simulink model "IEEE39_IBR_FrequencyControl_Fullversion_2020a"  (R2020a)
settings: Solver=VariableStepAuto  StartTime=0.0  StopTime=30  RelTol=1e-3
InitFcn:
  | IEEE39data_FrencyControl_full_Opensource;
undefined symbols (not defined in the file): alpha, c, eps_ps, eps_u, Fref, IBR_data, line, Sbase, t_start_disturbance, t_startcontrol, Vbase
libraries: powerlib x202, powerlib_meascontrol x81, powerlib_extras x27, simulink x18
(part 4 of 5)

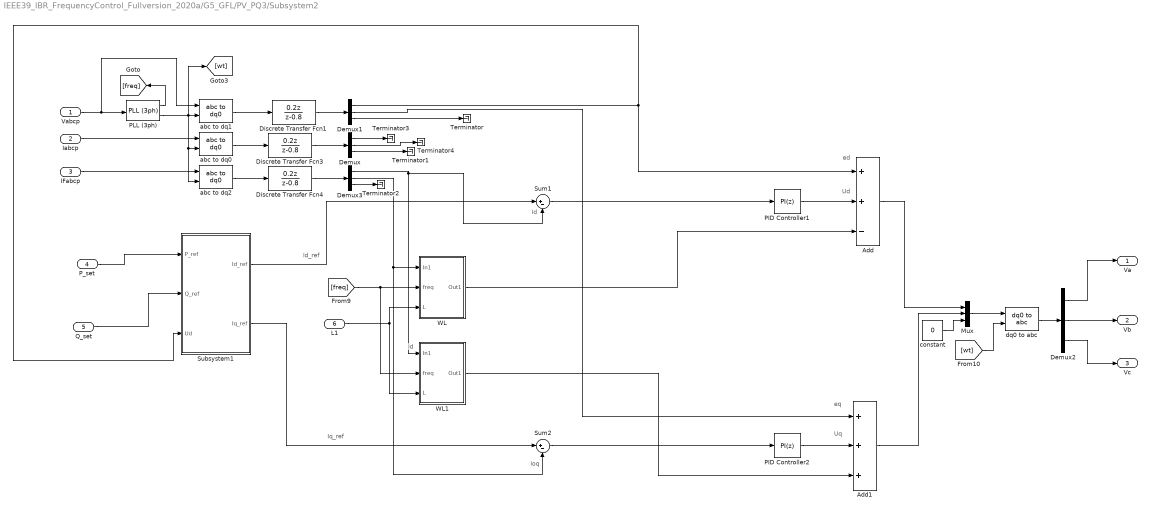
== system IEEE39_IBR_FrequencyControl_Fullversion_2020a/G5_GFL/PV_PQ3/Subsystem2 ==
  note: Iq_ref
  note: Id
  note: Id_ref
  note: Ud
  note: Uq
  note: eq
  note: ed
  note: Ioq
  note: Id
  Vabcp : Inport
  Iabcp : Inport  Port=2
  IFabcp : Inport  Port=3
  P_set : Inport  Port=4
  Q_set : Inport  Port=5
  L1 : Inport  Port=6
  Add : Sum  Inputs=++-
  Add1 : Sum  Inputs=+++
  Demux{,1..3} (4 alike) : Demux  Outputs=3
  Discrete Transfer Fcn1 : DiscreteTransferFcn  Numerator=[0.2 0]  Denominator=[1 -0.8]  InitialStates=[1 1 1]  SampleTime=5e-4
  Discrete Transfer Fcn3 : DiscreteTransferFcn  Numerator=[0.2 0]  Denominator=[1 -0.8]  SampleTime=5e-4
  Discrete Transfer Fcn4 : DiscreteTransferFcn  Numerator=[0.2 0]  Denominator=[1 -0.8]  SampleTime=5e-4
  Mux : Mux  Inputs=3
  PID Controller1 : simulink/Continuous/PID Controller  Controller=PI  Form=Parallel  TimeDomain=Discrete-time  UseExternalTs=off  SampleTime=5e-4  IntegratorMethod=Forward Euler  ControllerParametersSource=internal  P=100  I=400  D=0  N=100  UseFilter=on  TunerSelectOption=Transfer Function Based (PID Tuner App)  InitialConditionSource=internal  InitialConditionForIntegrator=0  InitialConditionForFilter=0  DifferentiatorICPrevScaledInput=0  ExternalReset=none  TrackingMode=off  Kt=1  LimitOutput=off  UpperSaturationLimit=inf  LowerSaturationLimit=-inf  LinearizeAsGain=on  AntiWindupMode=none  Kb=1  POutMin=[]  POutMax=[]  IOutMin=[]  IOutMax=[]  DOutMin=[]  DOutMax=[]  NOutMin=[]  NOutMax=[]  SumOutMin=[]  SumOutMax=[]  SaturationOutMin=[]  SaturationOutMax=[]  PParamMin=[]  PParamMax=[]  IParamMin=[]  IParamMax=[]  DParamMin=[]  DParamMax=[]  NParamMin=[]  NParamMax=[]  KbParamMin=[]  KbParamMax=[]  KtParamMin=[]  KtParamMax=[]  KbOutMin=[]  KbOutMax=[]  KtOutMin=[]  KtOutMax=[]  IntegratorOutMin=[]  IntegratorOutMax=[]  FilterOutMin=[]  FilterOutMax=[]  SumI1OutMin=[]  SumI1OutMax=[]  SumI2OutMin=[]  SumI2OutMax=[]  SumI3OutMin=[]  SumI3OutMax=[]  SumI4OutMin=[]  SumI4OutMax=[]  SumDOutMin=[]  SumDOutMax=[]  DifferentiatorOutMin=[]  DifferentiatorOutMax=[]  FilterDiffOutCoefMin=[]  FilterDiffOutCoefMax=[]  ReciprocalOutMin=[]  ReciprocalOutMax=[]  SumDenOutMin=[]  SumDenOutMax=[]  SumNumOutMin=[]  SumNumOutMax=[]  DivideOutMin=[]  DivideOutMax=[]  UdiffTsProdOutMin=[]  UdiffTsProdOutMax=[]  NTsProdOutMin=[]  NTsProdOutMax=[]  UintegralTsProdOutMin=[]  UintegralTsProdOutMax=[]  UngainTsProdOutMin=[]  UngainTsProdOutMax=[]  IntegratorContinuousStateAttributes=''  IntegratorStateMustResolveToSignalObject=off  IntegratorRTWStateStorageClass=Auto  FilterContinuousStateAttributes=''  FilterStateMustResolveToSignalObject=off  FilterRTWStateStorageClass=Auto  ParallelPVariant=InternalParameters  IdealPVariant=Disabled  IVariant=InternalParameters  DVariant=Disabled  IntegratorVariant=Discrete  SatVariant=Disabled  AWVariant=Passthrough  PCopyVariant=Disabled  TRVariant=Disabled  FdbkBlocksVariant=Forward  IdealPFdbkVariant=Disabled  SatFdbkVariant=Disabled  DerivativeFilterVariant=Disabled  NVariant=Disabled  NCopyVariant=Disabled_SignalSpec  FilterICVariant=Disabled  IntegratorICVariant=InternalICs  ExternalResetVariant=Disabled  TRSumVariant=Passthrough  SumFdbkVariant=Disabled  SumVariant=Sum_PI  TsampFilterVariant=InternalTs  TsampNgainVariant=Passthrough  TsampIntegralVariant=Disabled_SignalSpec
  PID Controller2 : simulink/Continuous/PID Controller  Controller=PI  Form=Parallel  TimeDomain=Discrete-time  UseExternalTs=off  SampleTime=5e-4  IntegratorMethod=Forward Euler  ControllerParametersSource=internal  P=100  I=400  D=0  N=100  UseFilter=on  TunerSelectOption=Transfer Function Based (PID Tuner App)  InitialConditionSource=internal  InitialConditionForIntegrator=0  InitialConditionForFilter=0  DifferentiatorICPrevScaledInput=0  ExternalReset=none  TrackingMode=off  Kt=1  LimitOutput=off  UpperSaturationLimit=inf  LowerSaturationLimit=-inf  LinearizeAsGain=on  AntiWindupMode=none  Kb=1  POutMin=[]  POutMax=[]  IOutMin=[]  IOutMax=[]  DOutMin=[]  DOutMax=[]  NOutMin=[]  NOutMax=[]  SumOutMin=[]  SumOutMax=[]  SaturationOutMin=[]  SaturationOutMax=[]  PParamMin=[]  PParamMax=[]  IParamMin=[]  IParamMax=[]  DParamMin=[]  DParamMax=[]  NParamMin=[]  NParamMax=[]  KbParamMin=[]  KbParamMax=[]  KtParamMin=[]  KtParamMax=[]  KbOutMin=[]  KbOutMax=[]  KtOutMin=[]  KtOutMax=[]  IntegratorOutMin=[]  IntegratorOutMax=[]  FilterOutMin=[]  FilterOutMax=[]  SumI1OutMin=[]  SumI1OutMax=[]  SumI2OutMin=[]  SumI2OutMax=[]  SumI3OutMin=[]  SumI3OutMax=[]  SumI4OutMin=[]  SumI4OutMax=[]  SumDOutMin=[]  SumDOutMax=[]  DifferentiatorOutMin=[]  DifferentiatorOutMax=[]  FilterDiffOutCoefMin=[]  FilterDiffOutCoefMax=[]  ReciprocalOutMin=[]  ReciprocalOutMax=[]  SumDenOutMin=[]  SumDenOutMax=[]  SumNumOutMin=[]  SumNumOutMax=[]  DivideOutMin=[]  DivideOutMax=[]  UdiffTsProdOutMin=[]  UdiffTsProdOutMax=[]  NTsProdOutMin=[]  NTsProdOutMax=[]  UintegralTsProdOutMin=[]  UintegralTsProdOutMax=[]  UngainTsProdOutMin=[]  UngainTsProdOutMax=[]  IntegratorContinuousStateAttributes=''  IntegratorStateMustResolveToSignalObject=off  IntegratorRTWStateStorageClass=Auto  FilterContinuousStateAttributes=''  FilterStateMustResolveToSignalObject=off  FilterRTWStateStorageClass=Auto  ParallelPVariant=InternalParameters  IdealPVariant=Disabled  IVariant=InternalParameters  DVariant=Disabled  IntegratorVariant=Discrete  SatVariant=Disabled  AWVariant=Passthrough  PCopyVariant=Disabled  TRVariant=Disabled  FdbkBlocksVariant=Forward  IdealPFdbkVariant=Disabled  SatFdbkVariant=Disabled  DerivativeFilterVariant=Disabled  NVariant=Disabled  NCopyVariant=Disabled_SignalSpec  FilterICVariant=Disabled  IntegratorICVariant=InternalICs  ExternalResetVariant=Disabled  TRSumVariant=Passthrough  SumFdbkVariant=Disabled  SumVariant=Sum_PI  TsampFilterVariant=InternalTs  TsampNgainVariant=Passthrough  TsampIntegralVariant=Disabled_SignalSpec
  PLL (3ph) : powerlib_meascontrol/PLL/PLL (3ph)  Fmin=59.5  Par_Init=[0, 60]  ParK=[180, 3200, 1]  TcD=1e-4  MaxRateChangeFreq=12  FilterCutOffFreq=25  Ts=1e-5  AGC=on
  Subsystem1 : Subsystem
  Sum1 : Sum  Inputs=|+-
  Sum2 : Sum  Inputs=|+-
  Terminator{,1..4} (5 alike) : Terminator
  WL : Subsystem
  WL1 : Subsystem
  abc to dq0 : powerlib_meascontrol/Transformations/abc to dq0  Alignment=90 degrees behind phase A axis
  abc to dq1 : powerlib_meascontrol/Transformations/abc to dq0  Alignment=90 degrees behind phase A axis
  abc to dq2 : powerlib_meascontrol/Transformations/abc to dq0  Alignment=90 degrees behind phase A axis
  constant : Constant  Value=0
  dq0 to abc : powerlib_meascontrol/Transformations/dq0 to abc  Alignment=90 degrees behind phase A axis
  Va : Outport  VectorParamsAs1DForOutWhenUnconnected=off
  Vb : Outport  Port=2  VectorParamsAs1DForOutWhenUnconnected=off
  Vc : Outport  Port=3  VectorParamsAs1DForOutWhenUnconnected=off
  wires:
  abc to dq0/1 -> Discrete Transfer Fcn3/1
  PLL (3ph)/2 -> [wt], abc to dq1/2, abc to dq2/2, abc to dq0/2
  Demux1/1 -> Add/1, Subsystem1/3(Ud)
  L1/1 -> WL/3(L), WL1/3(L)
  WL/1(Out1) -> Add/3
  [freq] -> WL1/2(freq), WL/2(freq)
  PLL (3ph)/1 -> [freq]
  Demux2/1 -> Va/1
  Add/1 -> Mux/1
  PID Controller2/1 -> Add1/2
  Demux2/2 -> Vb/1
  WL1/1(Out1) -> Add1/3
  Demux1/2 -> Add1/1
  Add1/1 -> Mux/2
  Mux/1 -> dq0 to abc/1
  Demux2/3 -> Vc/1
  dq0 to abc/1 -> Demux2/1
  Subsystem1/1(Id_ref) -> Sum1/1
  PID Controller1/1 -> Add/2
  [wt] -> dq0 to abc/2
  Subsystem1/2(Iq_ref) -> Sum2/1
  Demux1/3 -> Terminator/1
  Demux/3 -> Terminator1/1
  constant/1 -> Mux/3
  IFabcp/1 -> abc to dq2/1
  abc to dq2/1 -> Discrete Transfer Fcn4/1
  Demux3/3 -> Terminator2/1
  Demux3/2 -> Sum2/2, WL/1(In1)
  Demux3/1 -> Sum1/2, WL1/1(In1)
  Sum1/1 -> PID Controller1/1
  Sum2/1 -> PID Controller2/1
  P_set/1 -> Subsystem1/1(P_ref)
  Q_set/1 -> Subsystem1/2(Q_ref)
  Discrete Transfer Fcn3/1 -> Demux/1
  Discrete Transfer Fcn4/1 -> Demux3/1
  Demux/1 -> Terminator3/1
  Demux/2 -> Terminator4/1
  Discrete Transfer Fcn1/1 -> Demux1/1
  Iabcp/1 -> abc to dq0/1
  Vabcp/1 -> abc to dq1/1, PLL (3ph)/1
  abc to dq1/1 -> Discrete Transfer Fcn1/1

== system IEEE39_IBR_FrequencyControl_Fullversion_2020a/G6_GFL/PV_PQ3/Freq_Droop ==
  Pref : Inport
  Fref : Inport  Port=2
  Freq : Inport  Port=3
  D : Inport  Port=4
  Clock : Clock
  Constant : Constant  Value=0
  Divide : Product  Inputs=*/
  Product{,1..3} (4 alike) : Product
  S_base : Constant  Value=Sbase
  S_base1 : Constant  Value=Sbase
  Saturation : Saturate  UpperLimit=10*Sbase  LowerLimit=0  ZeroCross=off
  Subsystem : Subsystem
  Sum : Sum  Inputs=|+-
  Sum1 : Sum  Inputs=|+--
  Switch : Switch  Criteria=u2 > Threshold  Threshold=t_startcontrol  ZeroCross=off
  Transfer Fcn : TransferFcn  Denominator=[0.318 1]
  Pset : Outport
  tag scope: deltaP6=global
  wires:
  Freq/1 -> Sum/1
  Fref/1 -> Sum/2, Divide/2
  S_base/1 -> Product/2
  D/1 -> Product2/1, Product1/1
  Product/1 -> Product1/2
  Pref/1 -> Sum1/1
  Product1/1 -> Sum1/2
  Saturation/1 -> Pset/1
  Sum1/1 -> Saturation/1
  Subsystem/1(delatPset) -> Switch/1
  Clock/1 -> Switch/2
  Sum/1 -> Divide/1
  Constant/1 -> Switch/3
  Product2/1 -> Subsystem/1(Dw)
  Switch/1 -> [deltaP6], Product3/1
  S_base1/1 -> Product3/2
  Product3/1 -> Sum1/3
  Transfer Fcn/1 -> Subsystem/2(w), Product2/2, Product/1
  Divide/1 -> Transfer Fcn/1

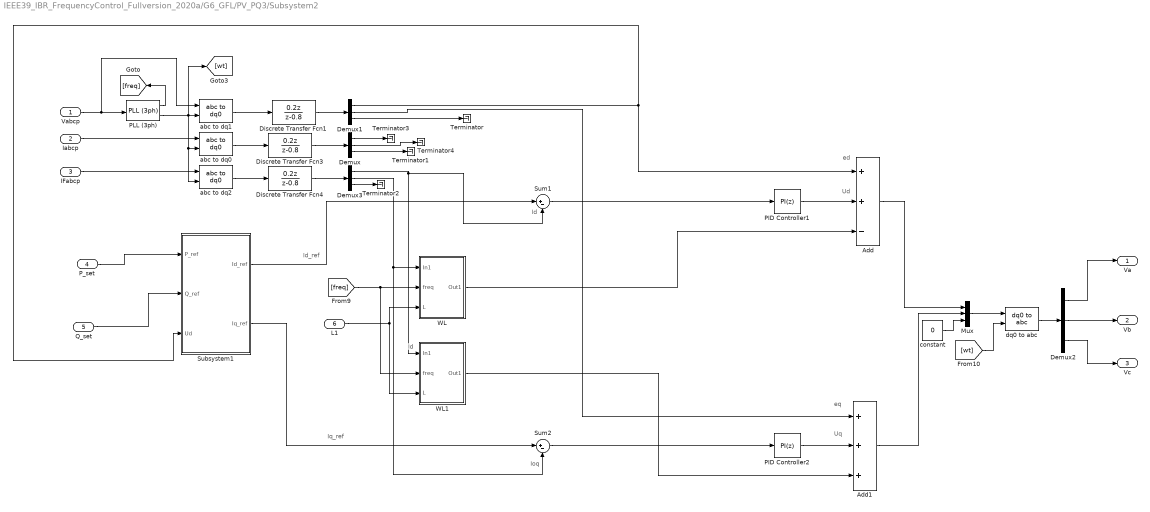
== system IEEE39_IBR_FrequencyControl_Fullversion_2020a/G6_GFL/PV_PQ3/Subsystem2 ==
  note: Iq_ref
  note: Id
  note: Id_ref
  note: Ud
  note: Uq
  note: eq
  note: ed
  note: Ioq
  note: Id
  Vabcp : Inport
  Iabcp : Inport  Port=2
  IFabcp : Inport  Port=3
  P_set : Inport  Port=4
  Q_set : Inport  Port=5
  L1 : Inport  Port=6
  Add : Sum  Inputs=++-
  Add1 : Sum  Inputs=+++
  Demux{,1..3} (4 alike) : Demux  Outputs=3
  Discrete Transfer Fcn1 : DiscreteTransferFcn  Numerator=[0.2 0]  Denominator=[1 -0.8]  InitialStates=[1 1 1]  SampleTime=5e-4
  Discrete Transfer Fcn3 : DiscreteTransferFcn  Numerator=[0.2 0]  Denominator=[1 -0.8]  SampleTime=5e-4
  Discrete Transfer Fcn4 : DiscreteTransferFcn  Numerator=[0.2 0]  Denominator=[1 -0.8]  SampleTime=5e-4
  Mux : Mux  Inputs=3
  PID Controller1 : simulink/Continuous/PID Controller  Controller=PI  Form=Parallel  TimeDomain=Discrete-time  UseExternalTs=off  SampleTime=5e-4  IntegratorMethod=Forward Euler  ControllerParametersSource=internal  P=50  I=400  D=0  N=100  UseFilter=on  TunerSelectOption=Transfer Function Based (PID Tuner App)  InitialConditionSource=internal  InitialConditionForIntegrator=0  InitialConditionForFilter=0  DifferentiatorICPrevScaledInput=0  ExternalReset=none  TrackingMode=off  Kt=1  LimitOutput=off  UpperSaturationLimit=inf  LowerSaturationLimit=-inf  LinearizeAsGain=on  AntiWindupMode=none  Kb=1  POutMin=[]  POutMax=[]  IOutMin=[]  IOutMax=[]  DOutMin=[]  DOutMax=[]  NOutMin=[]  NOutMax=[]  SumOutMin=[]  SumOutMax=[]  SaturationOutMin=[]  SaturationOutMax=[]  PParamMin=[]  PParamMax=[]  IParamMin=[]  IParamMax=[]  DParamMin=[]  DParamMax=[]  NParamMin=[]  NParamMax=[]  KbParamMin=[]  KbParamMax=[]  KtParamMin=[]  KtParamMax=[]  KbOutMin=[]  KbOutMax=[]  KtOutMin=[]  KtOutMax=[]  IntegratorOutMin=[]  IntegratorOutMax=[]  FilterOutMin=[]  FilterOutMax=[]  SumI1OutMin=[]  SumI1OutMax=[]  SumI2OutMin=[]  SumI2OutMax=[]  SumI3OutMin=[]  SumI3OutMax=[]  SumI4OutMin=[]  SumI4OutMax=[]  SumDOutMin=[]  SumDOutMax=[]  DifferentiatorOutMin=[]  DifferentiatorOutMax=[]  FilterDiffOutCoefMin=[]  FilterDiffOutCoefMax=[]  ReciprocalOutMin=[]  ReciprocalOutMax=[]  SumDenOutMin=[]  SumDenOutMax=[]  SumNumOutMin=[]  SumNumOutMax=[]  DivideOutMin=[]  DivideOutMax=[]  UdiffTsProdOutMin=[]  UdiffTsProdOutMax=[]  NTsProdOutMin=[]  NTsProdOutMax=[]  UintegralTsProdOutMin=[]  UintegralTsProdOutMax=[]  UngainTsProdOutMin=[]  UngainTsProdOutMax=[]  IntegratorContinuousStateAttributes=''  IntegratorStateMustResolveToSignalObject=off  IntegratorRTWStateStorageClass=Auto  FilterContinuousStateAttributes=''  FilterStateMustResolveToSignalObject=off  FilterRTWStateStorageClass=Auto  ParallelPVariant=InternalParameters  IdealPVariant=Disabled  IVariant=InternalParameters  DVariant=Disabled  IntegratorVariant=Discrete  SatVariant=Disabled  AWVariant=Passthrough  PCopyVariant=Disabled  TRVariant=Disabled  FdbkBlocksVariant=Forward  IdealPFdbkVariant=Disabled  SatFdbkVariant=Disabled  DerivativeFilterVariant=Disabled  NVariant=Disabled  NCopyVariant=Disabled_SignalSpec  FilterICVariant=Disabled  IntegratorICVariant=InternalICs  ExternalResetVariant=Disabled  TRSumVariant=Passthrough  SumFdbkVariant=Disabled  SumVariant=Sum_PI  TsampFilterVariant=InternalTs  TsampNgainVariant=Passthrough  TsampIntegralVariant=Disabled_SignalSpec
  PID Controller2 : simulink/Continuous/PID Controller  Controller=PI  Form=Parallel  TimeDomain=Discrete-time  UseExternalTs=off  SampleTime=5e-4  IntegratorMethod=Forward Euler  ControllerParametersSource=internal  P=50  I=400  D=0  N=100  UseFilter=on  TunerSelectOption=Transfer Function Based (PID Tuner App)  InitialConditionSource=internal  InitialConditionForIntegrator=0  InitialConditionForFilter=0  DifferentiatorICPrevScaledInput=0  ExternalReset=none  TrackingMode=off  Kt=1  LimitOutput=off  UpperSaturationLimit=inf  LowerSaturationLimit=-inf  LinearizeAsGain=on  AntiWindupMode=none  Kb=1  POutMin=[]  POutMax=[]  IOutMin=[]  IOutMax=[]  DOutMin=[]  DOutMax=[]  NOutMin=[]  NOutMax=[]  SumOutMin=[]  SumOutMax=[]  SaturationOutMin=[]  SaturationOutMax=[]  PParamMin=[]  PParamMax=[]  IParamMin=[]  IParamMax=[]  DParamMin=[]  DParamMax=[]  NParamMin=[]  NParamMax=[]  KbParamMin=[]  KbParamMax=[]  KtParamMin=[]  KtParamMax=[]  KbOutMin=[]  KbOutMax=[]  KtOutMin=[]  KtOutMax=[]  IntegratorOutMin=[]  IntegratorOutMax=[]  FilterOutMin=[]  FilterOutMax=[]  SumI1OutMin=[]  SumI1OutMax=[]  SumI2OutMin=[]  SumI2OutMax=[]  SumI3OutMin=[]  SumI3OutMax=[]  SumI4OutMin=[]  SumI4OutMax=[]  SumDOutMin=[]  SumDOutMax=[]  DifferentiatorOutMin=[]  DifferentiatorOutMax=[]  FilterDiffOutCoefMin=[]  FilterDiffOutCoefMax=[]  ReciprocalOutMin=[]  ReciprocalOutMax=[]  SumDenOutMin=[]  SumDenOutMax=[]  SumNumOutMin=[]  SumNumOutMax=[]  DivideOutMin=[]  DivideOutMax=[]  UdiffTsProdOutMin=[]  UdiffTsProdOutMax=[]  NTsProdOutMin=[]  NTsProdOutMax=[]  UintegralTsProdOutMin=[]  UintegralTsProdOutMax=[]  UngainTsProdOutMin=[]  UngainTsProdOutMax=[]  IntegratorContinuousStateAttributes=''  IntegratorStateMustResolveToSignalObject=off  IntegratorRTWStateStorageClass=Auto  FilterContinuousStateAttributes=''  FilterStateMustResolveToSignalObject=off  FilterRTWStateStorageClass=Auto  ParallelPVariant=InternalParameters  IdealPVariant=Disabled  IVariant=InternalParameters  DVariant=Disabled  IntegratorVariant=Discrete  SatVariant=Disabled  AWVariant=Passthrough  PCopyVariant=Disabled  TRVariant=Disabled  FdbkBlocksVariant=Forward  IdealPFdbkVariant=Disabled  SatFdbkVariant=Disabled  DerivativeFilterVariant=Disabled  NVariant=Disabled  NCopyVariant=Disabled_SignalSpec  FilterICVariant=Disabled  IntegratorICVariant=InternalICs  ExternalResetVariant=Disabled  TRSumVariant=Passthrough  SumFdbkVariant=Disabled  SumVariant=Sum_PI  TsampFilterVariant=InternalTs  TsampNgainVariant=Passthrough  TsampIntegralVariant=Disabled_SignalSpec
  PLL (3ph) : powerlib_meascontrol/PLL/PLL (3ph)  Fmin=59.5  Par_Init=[0, 60]  ParK=[180, 3200, 1]  TcD=1e-4  MaxRateChangeFreq=12  FilterCutOffFreq=25  Ts=1e-5  AGC=on
  Subsystem1 : Subsystem
  Sum1 : Sum  Inputs=|+-
  Sum2 : Sum  Inputs=|+-
  Terminator{,1..4} (5 alike) : Terminator
  WL : Subsystem
  WL1 : Subsystem
  abc to dq0 : powerlib_meascontrol/Transformations/abc to dq0  Alignment=90 degrees behind phase A axis
  abc to dq1 : powerlib_meascontrol/Transformations/abc to dq0  Alignment=90 degrees behind phase A axis
  abc to dq2 : powerlib_meascontrol/Transformations/abc to dq0  Alignment=90 degrees behind phase A axis
  constant : Constant  Value=0
  dq0 to abc : powerlib_meascontrol/Transformations/dq0 to abc  Alignment=90 degrees behind phase A axis
  Va : Outport  VectorParamsAs1DForOutWhenUnconnected=off
  Vb : Outport  Port=2  VectorParamsAs1DForOutWhenUnconnected=off
  Vc : Outport  Port=3  VectorParamsAs1DForOutWhenUnconnected=off
  wires:
  abc to dq0/1 -> Discrete Transfer Fcn3/1
  PLL (3ph)/2 -> [wt], abc to dq1/2, abc to dq2/2, abc to dq0/2
  Demux1/1 -> Add/1, Subsystem1/3(Ud)
  L1/1 -> WL/3(L), WL1/3(L)
  WL/1(Out1) -> Add/3
  [freq] -> WL1/2(freq), WL/2(freq)
  PLL (3ph)/1 -> [freq]
  Demux2/1 -> Va/1
  Add/1 -> Mux/1
  PID Controller2/1 -> Add1/2
  Demux2/2 -> Vb/1
  WL1/1(Out1) -> Add1/3
  Demux1/2 -> Add1/1
  Add1/1 -> Mux/2
  Mux/1 -> dq0 to abc/1
  Demux2/3 -> Vc/1
  dq0 to abc/1 -> Demux2/1
  Subsystem1/1(Id_ref) -> Sum1/1
  PID Controller1/1 -> Add/2
  [wt] -> dq0 to abc/2
  Subsystem1/2(Iq_ref) -> Sum2/1
  Demux1/3 -> Terminator/1
  Demux/3 -> Terminator1/1
  constant/1 -> Mux/3
  IFabcp/1 -> abc to dq2/1
  abc to dq2/1 -> Discrete Transfer Fcn4/1
  Demux3/3 -> Terminator2/1
  Demux3/2 -> Sum2/2, WL/1(In1)
  Demux3/1 -> Sum1/2, WL1/1(In1)
  Sum1/1 -> PID Controller1/1
  Sum2/1 -> PID Controller2/1
  P_set/1 -> Subsystem1/1(P_ref)
  Q_set/1 -> Subsystem1/2(Q_ref)
  Discrete Transfer Fcn3/1 -> Demux/1
  Discrete Transfer Fcn4/1 -> Demux3/1
  Demux/1 -> Terminator3/1
  Demux/2 -> Terminator4/1
  Discrete Transfer Fcn1/1 -> Demux1/1
  Iabcp/1 -> abc to dq0/1
  Vabcp/1 -> abc to dq1/1, PLL (3ph)/1
  abc to dq1/1 -> Discrete Transfer Fcn1/1

== system IEEE39_IBR_FrequencyControl_Fullversion_2020a/GFM1/PV_PQ3/Freq_Droop ==
  Pref : Inport
  Fref : Inport  Port=2
  Pmeans : Inport  Port=3
  Add : Sum  Inputs=+-
  Add1 : Sum
  Add2 : Sum  Inputs=+-
  Add3 : Sum  Inputs=+-
  Divide : Product  Inputs=*/
  Divide2 : Product  Inputs=*/
  Product : Product
  S_base : Constant  Value=Sbase
  Saturation : Saturate  UpperLimit=2  LowerLimit=-2  ZeroCross=off
  Step : Step  Time=5  SampleTime=0
  Subsystem1 : Subsystem
  Switch : Switch  Criteria=u2 > Threshold
  Transfer Fcn : TransferFcn  Denominator=[IBR_data(10,5) IBR_data(10,4)]
  Transfer Fcn1 : TransferFcn  Numerator=[20]  Denominator=[1 20]
  Transfer Fcn2 : TransferFcn  Denominator=[IBR_data(10,5) IBR_data(10,4)]
  fset : Outport
  wires:
  Pref/1 -> Add/1
  Transfer Fcn1/1 -> Add/2
  S_base/1 -> Divide/2
  Switch/1 -> Product/1
  Add1/1 -> fset/1
  Saturation/1 -> Add1/1
  Product/1 -> Saturation/1
  Divide/1 -> Add3/1
  Add/1 -> Divide/1
  Pmeans/1 -> Transfer Fcn1/1
  [f10] -> Add2/1
  Fref/1 -> Add1/2, Divide2/2, Add2/2, Product/2
  Add2/1 -> Divide2/1
  Divide2/1 -> Subsystem1/1(w)
  Transfer Fcn2/1 -> Switch/1
  Transfer Fcn/1 -> Switch/3
  Step/1 -> Switch/2
  Add3/1 -> Transfer Fcn/1, Transfer Fcn2/1
  Subsystem1/1(Out1) -> Add3/2

== system IEEE39_IBR_FrequencyControl_Fullversion_2020a/GFM1/PV_PQ3/V//F ==
  vabcb : Inport
  iabcb : Inport  Port=2
  iFabcb : Inport  Port=3
  Vref_LL : Inport  Port=4
  f : Inport  Port=5
  Init_Phase_degree : Inport  Port=6
  Constant1 : Constant  Value=0
  Constant2 : Constant  Value=sqrt(2)/sqrt(3)
  Product : Product
  Subsystem : Subsystem
  UIcontrol : Subsystem
  Va : Outport
  Vb : Outport  Port=2
  Vc : Outport  Port=3
  wires:
  Constant1/1 -> UIcontrol/3(eq_ref)
  vabcb/1 -> Subsystem/1(eo)
  iFabcb/1 -> Subsystem/3(i)
  iabcb/1 -> Subsystem/2(io)
  Subsystem/1(eod) -> UIcontrol/2(ed)
  Subsystem/2(eoq) -> UIcontrol/4(eq)
  Subsystem/3(iod) -> UIcontrol/5(iod)
  Subsystem/4(ioq) -> UIcontrol/6(ioq)
  Subsystem/5(id) -> UIcontrol/7(id)
  Subsystem/6(iq) -> UIcontrol/8(iq)
  Subsystem/7(w) -> UIcontrol/9(w)
  UIcontrol/1(Va) -> Va/1
  UIcontrol/2(Vb) -> Vb/1
  UIcontrol/3(Vc) -> Vc/1
  f/1 -> Subsystem/4(f)
  Init_Phase_degree/1 -> Subsystem/5(Init_Phase_degree)
  Vref_LL/1 -> Product/1
  Product/1 -> UIcontrol/1(ed_ref)
  Constant2/1 -> Product/2
  Subsystem/8("wt ") -> UIcontrol/10("wt ")

== system IEEE39_IBR_FrequencyControl_Fullversion_2020a/GFM2/PV_PQ3/Freq_Droop ==
  Pref : Inport
  Fref : Inport  Port=2
  Pmeans : Inport  Port=3
  Add : Sum  Inputs=+-
  Add1 : Sum
  Add2 : Sum  Inputs=+-
  Add3 : Sum  Inputs=+-
  Divide : Product  Inputs=*/
  Divide2 : Product  Inputs=*/
  Product : Product
  S_base : Constant  Value=Sbase
  Saturation : Saturate  UpperLimit=2  LowerLimit=-2  ZeroCross=off
  Step : Step  Time=5  SampleTime=0
  Subsystem1 : Subsystem
  Switch : Switch  Criteria=u2 > Threshold
  Transfer Fcn : TransferFcn  Denominator=[IBR_data(9,5) IBR_data(9,4)]
  Transfer Fcn1 : TransferFcn  Numerator=[20]  Denominator=[1 20]
  Transfer Fcn2 : TransferFcn  Denominator=[IBR_data(9,5) IBR_data(9,4)]
  fset : Outport
  wires:
  Pref/1 -> Add/1
  Transfer Fcn1/1 -> Add/2
  S_base/1 -> Divide/2
  Switch/1 -> Product/1
  Add1/1 -> fset/1
  Saturation/1 -> Add1/1
  Product/1 -> Saturation/1
  Divide/1 -> Add3/1
  Add/1 -> Divide/1
  Pmeans/1 -> Transfer Fcn1/1
  [f9] -> Add2/1
  Fref/1 -> Add1/2, Divide2/2, Add2/2, Product/2
  Add2/1 -> Divide2/1
  Divide2/1 -> Subsystem1/1(w)
  Transfer Fcn2/1 -> Switch/1
  Transfer Fcn/1 -> Switch/3
  Step/1 -> Switch/2
  Add3/1 -> Transfer Fcn/1, Transfer Fcn2/1
  Subsystem1/1(Out1) -> Add3/2

== system IEEE39_IBR_FrequencyControl_Fullversion_2020a/GFM2/PV_PQ3/V//F ==
  vabcb : Inport
  iabcb : Inport  Port=2
  iFabcb : Inport  Port=3
  Vref_LL : Inport  Port=4
  f : Inport  Port=5
  Init_Phase_degree : Inport  Port=6
  Constant : Constant  Value=2*pi
  Constant1 : Constant  Value=0
  Constant2 : Constant  Value=sqrt(2)/sqrt(3)
  Divide : Product  Inputs=*/
  Product : Product
  Scope1 : Scope
  Subsystem : Subsystem
  UIcontrol : Subsystem
  Va : Outport
  Vb : Outport  Port=2
  Vc : Outport  Port=3
  wires:
  Constant1/1 -> UIcontrol/3(eq_ref)
  vabcb/1 -> Subsystem/1(eo)
  iFabcb/1 -> Subsystem/3(i)
  iabcb/1 -> Subsystem/2(io)
  Subsystem/1(eod) -> UIcontrol/2(ed)
  Subsystem/2(eoq) -> UIcontrol/4(eq)
  Subsystem/3(iod) -> UIcontrol/5(iod)
  Subsystem/4(ioq) -> UIcontrol/6(ioq)
  Subsystem/5(id) -> UIcontrol/7(id)
  Subsystem/6(iq) -> UIcontrol/8(iq)
  Subsystem/7(w) -> Divide/1, UIcontrol/9(w)
  UIcontrol/1(Va) -> Va/1
  UIcontrol/2(Vb) -> Vb/1
  UIcontrol/3(Vc) -> Vc/1
  f/1 -> Subsystem/4(f)
  Init_Phase_degree/1 -> Subsystem/5(Init_Phase_degree)
  Vref_LL/1 -> Product/1
  Product/1 -> UIcontrol/1(ed_ref)
  Constant2/1 -> Product/2
  Subsystem/8("wt ") -> UIcontrol/10("wt ")
  Constant/1 -> Divide/2
  Divide/1 -> Scope1/1

== system IEEE39_IBR_FrequencyControl_Fullversion_2020a/GFM3/PV_PQ3/Freq_Droop ==
  Pref : Inport
  Fref : Inport  Port=2
  Pmeans : Inport  Port=3
  Add : Sum  Inputs=+-
  Add1 : Sum
  Add2 : Sum  Inputs=+-
  Add3 : Sum  Inputs=+-
  Divide : Product  Inputs=*/
  Divide2 : Product  Inputs=*/
  Product : Product
  S_base : Constant  Value=Sbase
  Saturation : Saturate  UpperLimit=2  LowerLimit=-2  ZeroCross=off
  Step : Step  Time=5  SampleTime=0
  Subsystem1 : Subsystem
  Switch : Switch  Criteria=u2 > Threshold
  Transfer Fcn : TransferFcn  Denominator=[IBR_data(8,5) IBR_data(8,4)]
  Transfer Fcn1 : TransferFcn  Numerator=[20]  Denominator=[1 20]
  Transfer Fcn2 : TransferFcn  Denominator=[IBR_data(8,5) IBR_data(8,4)]
  fset : Outport
  wires:
  Pref/1 -> Add/1
  Transfer Fcn1/1 -> Add/2
  S_base/1 -> Divide/2
  Switch/1 -> Product/1
  Add1/1 -> fset/1
  Saturation/1 -> Add1/1
  Product/1 -> Saturation/1
  Divide/1 -> Add3/1
  Add/1 -> Divide/1
  Pmeans/1 -> Transfer Fcn1/1
  [f8] -> Add2/1
  Fref/1 -> Add1/2, Divide2/2, Add2/2, Product/2
  Add2/1 -> Divide2/1
  Divide2/1 -> Subsystem1/1(w)
  Transfer Fcn2/1 -> Switch/1
  Transfer Fcn/1 -> Switch/3
  Step/1 -> Switch/2
  Add3/1 -> Transfer Fcn/1, Transfer Fcn2/1
  Subsystem1/1(Out1) -> Add3/2

== system IEEE39_IBR_FrequencyControl_Fullversion_2020a/GFM3/PV_PQ3/V//F ==
  vabcb : Inport
  iabcb : Inport  Port=2
  iFabcb : Inport  Port=3
  Vref_LL : Inport  Port=4
  f : Inport  Port=5
  Init_Phase_degree : Inport  Port=6
  Constant : Constant  Value=2*pi
  Constant1 : Constant  Value=0
  Constant2 : Constant  Value=sqrt(2)/sqrt(3)
  Divide : Product  Inputs=*/
  Product : Product
  Scope1 : Scope
  Subsystem : Subsystem
  UIcontrol : Subsystem
  Va : Outport
  Vb : Outport  Port=2
  Vc : Outport  Port=3
  wires:
  Constant1/1 -> UIcontrol/3(eq_ref)
  vabcb/1 -> Subsystem/1(eo)
  iFabcb/1 -> Subsystem/3(i)
  iabcb/1 -> Subsystem/2(io)
  Subsystem/1(eod) -> UIcontrol/2(ed)
  Subsystem/2(eoq) -> UIcontrol/4(eq)
  Subsystem/3(iod) -> UIcontrol/5(iod)
  Subsystem/4(ioq) -> UIcontrol/6(ioq)
  Subsystem/5(id) -> UIcontrol/7(id)
  Subsystem/6(iq) -> UIcontrol/8(iq)
  Subsystem/7(w) -> Divide/1, UIcontrol/9(w)
  UIcontrol/1(Va) -> Va/1
  UIcontrol/2(Vb) -> Vb/1
  UIcontrol/3(Vc) -> Vc/1
  f/1 -> Subsystem/4(f)
  Init_Phase_degree/1 -> Subsystem/5(Init_Phase_degree)
  Vref_LL/1 -> Product/1
  Product/1 -> UIcontrol/1(ed_ref)
  Constant2/1 -> Product/2
  Subsystem/8("wt ") -> UIcontrol/10("wt ")
  Constant/1 -> Divide/2
  Divide/1 -> Scope1/1

== system IEEE39_IBR_FrequencyControl_Fullversion_2020a/GFM4/PV_PQ3/Freq_Droop ==
  Pref : Inport
  Fref : Inport  Port=2
  Pmeans : Inport  Port=3
  Add : Sum  Inputs=+-
  Add1 : Sum
  Add2 : Sum  Inputs=+-
  Add3 : Sum  Inputs=+-
  Divide : Product  Inputs=*/
  Divide2 : Product  Inputs=*/
  Product : Product
  S_base : Constant  Value=Sbase
  Saturation : Saturate  UpperLimit=2  LowerLimit=-2  ZeroCross=off
  Step : Step  Time=5  SampleTime=0
  Subsystem1 : Subsystem
  Switch : Switch  Criteria=u2 > Threshold
  Transfer Fcn : TransferFcn  Denominator=[IBR_data(7,5) IBR_data(7,4)]
  Transfer Fcn1 : TransferFcn  Numerator=[20]  Denominator=[1 20]
  Transfer Fcn2 : TransferFcn  Denominator=[IBR_data(7,5) IBR_data(7,4)]
  fset : Outport
  wires:
  Pref/1 -> Add/1
  Transfer Fcn1/1 -> Add/2
  S_base/1 -> Divide/2
  Switch/1 -> Product/1
  Add1/1 -> fset/1
  Saturation/1 -> Add1/1
  Product/1 -> Saturation/1
  Divide/1 -> Add3/1
  Add/1 -> Divide/1
  Pmeans/1 -> Transfer Fcn1/1
  [f8] -> Add2/1
  Fref/1 -> Add1/2, Divide2/2, Add2/2, Product/2
  Add2/1 -> Divide2/1
  Divide2/1 -> Subsystem1/1(w)
  Transfer Fcn2/1 -> Switch/1
  Transfer Fcn/1 -> Switch/3
  Step/1 -> Switch/2
  Add3/1 -> Transfer Fcn/1, Transfer Fcn2/1
  Subsystem1/1(Out1) -> Add3/2

== system IEEE39_IBR_FrequencyControl_Fullversion_2020a/GFM4/PV_PQ3/V//F ==
  vabcb : Inport
  iabcb : Inport  Port=2
  iFabcb : Inport  Port=3
  Vref_LL : Inport  Port=4
  f : Inport  Port=5
  Init_Phase_degree : Inport  Port=6
  Constant : Constant  Value=2*pi
  Constant1 : Constant  Value=0
  Constant2 : Constant  Value=sqrt(2)/sqrt(3)
  Divide : Product  Inputs=*/
  Product : Product
  Scope1 : Scope
  Subsystem : Subsystem
  UIcontrol : Subsystem
  Va : Outport
  Vb : Outport  Port=2
  Vc : Outport  Port=3
  wires:
  Constant1/1 -> UIcontrol/3(eq_ref)
  vabcb/1 -> Subsystem/1(eo)
  iFabcb/1 -> Subsystem/3(i)
  iabcb/1 -> Subsystem/2(io)
  Subsystem/1(eod) -> UIcontrol/2(ed)
  Subsystem/2(eoq) -> UIcontrol/4(eq)
  Subsystem/3(iod) -> UIcontrol/5(iod)
  Subsystem/4(ioq) -> UIcontrol/6(ioq)
  Subsystem/5(id) -> UIcontrol/7(id)
  Subsystem/6(iq) -> UIcontrol/8(iq)
  Subsystem/7(w) -> Divide/1, UIcontrol/9(w)
  UIcontrol/1(Va) -> Va/1
  UIcontrol/2(Vb) -> Vb/1
  UIcontrol/3(Vc) -> Vc/1
  f/1 -> Subsystem/4(f)
  Init_Phase_degree/1 -> Subsystem/5(Init_Phase_degree)
  Vref_LL/1 -> Product/1
  Product/1 -> UIcontrol/1(ed_ref)
  Constant2/1 -> Product/2
  Subsystem/8("wt ") -> UIcontrol/10("wt ")
  Constant/1 -> Divide/2
  Divide/1 -> Scope1/1

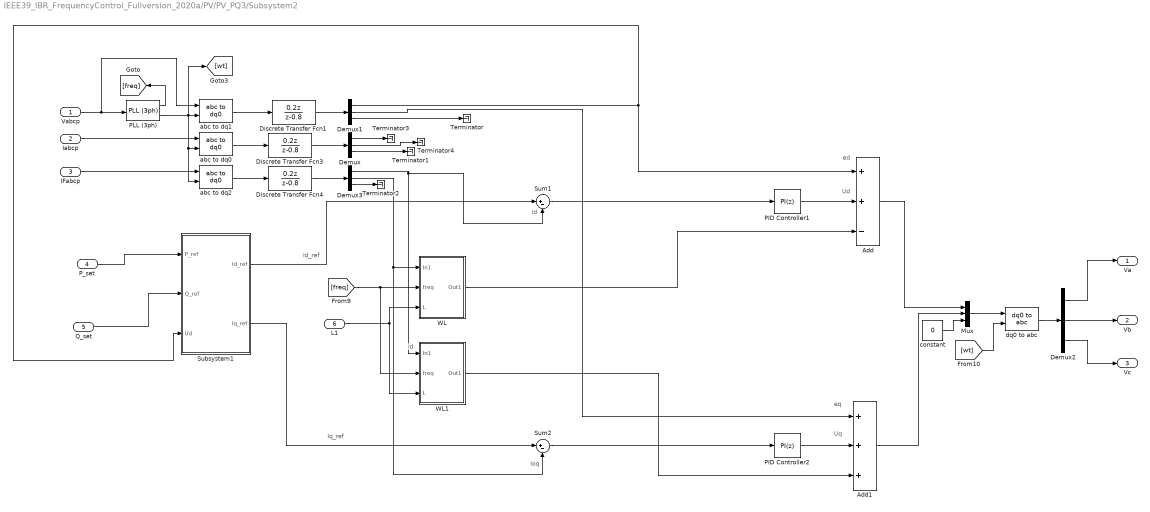
== system IEEE39_IBR_FrequencyControl_Fullversion_2020a/PV/PV_PQ3/Subsystem2 ==
  note: Iq_ref
  note: Id
  note: Id_ref
  note: Ud
  note: Uq
  note: eq
  note: ed
  note: Ioq
  note: Id
  Vabcp : Inport
  Iabcp : Inport  Port=2
  IFabcp : Inport  Port=3
  P_set : Inport  Port=4
  Q_set : Inport  Port=5
  L1 : Inport  Port=6
  Add : Sum  Inputs=++-
  Add1 : Sum  Inputs=+++
  Demux{,1..3} (4 alike) : Demux  Outputs=3
  Discrete Transfer Fcn1 : DiscreteTransferFcn  Numerator=[0.2 0]  Denominator=[1 -0.8]  InitialStates=[1 1 1]  SampleTime=5e-4
  Discrete Transfer Fcn3 : DiscreteTransferFcn  Numerator=[0.2 0]  Denominator=[1 -0.8]  SampleTime=5e-4
  Discrete Transfer Fcn4 : DiscreteTransferFcn  Numerator=[0.2 0]  Denominator=[1 -0.8]  SampleTime=5e-4
  Mux : Mux  Inputs=3
  PID Controller1 : simulink/Continuous/PID Controller  Controller=PI  Form=Parallel  TimeDomain=Discrete-time  UseExternalTs=off  SampleTime=5e-4  IntegratorMethod=Forward Euler  ControllerParametersSource=internal  P=100  I=400  D=0  N=100  UseFilter=on  TunerSelectOption=Transfer Function Based (PID Tuner App)  InitialConditionSource=internal  InitialConditionForIntegrator=0  InitialConditionForFilter=0  DifferentiatorICPrevScaledInput=0  ExternalReset=none  TrackingMode=off  Kt=1  LimitOutput=off  UpperSaturationLimit=inf  LowerSaturationLimit=-inf  LinearizeAsGain=on  AntiWindupMode=none  Kb=1  POutMin=[]  POutMax=[]  IOutMin=[]  IOutMax=[]  DOutMin=[]  DOutMax=[]  NOutMin=[]  NOutMax=[]  SumOutMin=[]  SumOutMax=[]  SaturationOutMin=[]  SaturationOutMax=[]  PParamMin=[]  PParamMax=[]  IParamMin=[]  IParamMax=[]  DParamMin=[]  DParamMax=[]  NParamMin=[]  NParamMax=[]  KbParamMin=[]  KbParamMax=[]  KtParamMin=[]  KtParamMax=[]  KbOutMin=[]  KbOutMax=[]  KtOutMin=[]  KtOutMax=[]  IntegratorOutMin=[]  IntegratorOutMax=[]  FilterOutMin=[]  FilterOutMax=[]  SumI1OutMin=[]  SumI1OutMax=[]  SumI2OutMin=[]  SumI2OutMax=[]  SumI3OutMin=[]  SumI3OutMax=[]  SumI4OutMin=[]  SumI4OutMax=[]  SumDOutMin=[]  SumDOutMax=[]  DifferentiatorOutMin=[]  DifferentiatorOutMax=[]  FilterDiffOutCoefMin=[]  FilterDiffOutCoefMax=[]  ReciprocalOutMin=[]  ReciprocalOutMax=[]  SumDenOutMin=[]  SumDenOutMax=[]  SumNumOutMin=[]  SumNumOutMax=[]  DivideOutMin=[]  DivideOutMax=[]  UdiffTsProdOutMin=[]  UdiffTsProdOutMax=[]  NTsProdOutMin=[]  NTsProdOutMax=[]  UintegralTsProdOutMin=[]  UintegralTsProdOutMax=[]  UngainTsProdOutMin=[]  UngainTsProdOutMax=[]  IntegratorContinuousStateAttributes=''  IntegratorStateMustResolveToSignalObject=off  IntegratorRTWStateStorageClass=Auto  FilterContinuousStateAttributes=''  FilterStateMustResolveToSignalObject=off  FilterRTWStateStorageClass=Auto  ParallelPVariant=InternalParameters  IdealPVariant=Disabled  IVariant=InternalParameters  DVariant=Disabled  IntegratorVariant=Discrete  SatVariant=Disabled  AWVariant=Passthrough  PCopyVariant=Disabled  TRVariant=Disabled  FdbkBlocksVariant=Forward  IdealPFdbkVariant=Disabled  SatFdbkVariant=Disabled  DerivativeFilterVariant=Disabled  NVariant=Disabled  NCopyVariant=Disabled_SignalSpec  FilterICVariant=Disabled  IntegratorICVariant=InternalICs  ExternalResetVariant=Disabled  TRSumVariant=Passthrough  SumFdbkVariant=Disabled  SumVariant=Sum_PI  TsampFilterVariant=InternalTs  TsampNgainVariant=Passthrough  TsampIntegralVariant=Disabled_SignalSpec
  PID Controller2 : simulink/Continuous/PID Controller  Controller=PI  Form=Parallel  TimeDomain=Discrete-time  UseExternalTs=off  SampleTime=5e-4  IntegratorMethod=Forward Euler  ControllerParametersSource=internal  P=100  I=400  D=0  N=100  UseFilter=on  TunerSelectOption=Transfer Function Based (PID Tuner App)  InitialConditionSource=internal  InitialConditionForIntegrator=0  InitialConditionForFilter=0  DifferentiatorICPrevScaledInput=0  ExternalReset=none  TrackingMode=off  Kt=1  LimitOutput=off  UpperSaturationLimit=inf  LowerSaturationLimit=-inf  LinearizeAsGain=on  AntiWindupMode=none  Kb=1  POutMin=[]  POutMax=[]  IOutMin=[]  IOutMax=[]  DOutMin=[]  DOutMax=[]  NOutMin=[]  NOutMax=[]  SumOutMin=[]  SumOutMax=[]  SaturationOutMin=[]  SaturationOutMax=[]  PParamMin=[]  PParamMax=[]  IParamMin=[]  IParamMax=[]  DParamMin=[]  DParamMax=[]  NParamMin=[]  NParamMax=[]  KbParamMin=[]  KbParamMax=[]  KtParamMin=[]  KtParamMax=[]  KbOutMin=[]  KbOutMax=[]  KtOutMin=[]  KtOutMax=[]  IntegratorOutMin=[]  IntegratorOutMax=[]  FilterOutMin=[]  FilterOutMax=[]  SumI1OutMin=[]  SumI1OutMax=[]  SumI2OutMin=[]  SumI2OutMax=[]  SumI3OutMin=[]  SumI3OutMax=[]  SumI4OutMin=[]  SumI4OutMax=[]  SumDOutMin=[]  SumDOutMax=[]  DifferentiatorOutMin=[]  DifferentiatorOutMax=[]  FilterDiffOutCoefMin=[]  FilterDiffOutCoefMax=[]  ReciprocalOutMin=[]  ReciprocalOutMax=[]  SumDenOutMin=[]  SumDenOutMax=[]  SumNumOutMin=[]  SumNumOutMax=[]  DivideOutMin=[]  DivideOutMax=[]  UdiffTsProdOutMin=[]  UdiffTsProdOutMax=[]  NTsProdOutMin=[]  NTsProdOutMax=[]  UintegralTsProdOutMin=[]  UintegralTsProdOutMax=[]  UngainTsProdOutMin=[]  UngainTsProdOutMax=[]  IntegratorContinuousStateAttributes=''  IntegratorStateMustResolveToSignalObject=off  IntegratorRTWStateStorageClass=Auto  FilterContinuousStateAttributes=''  FilterStateMustResolveToSignalObject=off  FilterRTWStateStorageClass=Auto  ParallelPVariant=InternalParameters  IdealPVariant=Disabled  IVariant=InternalParameters  DVariant=Disabled  IntegratorVariant=Discrete  SatVariant=Disabled  AWVariant=Passthrough  PCopyVariant=Disabled  TRVariant=Disabled  FdbkBlocksVariant=Forward  IdealPFdbkVariant=Disabled  SatFdbkVariant=Disabled  DerivativeFilterVariant=Disabled  NVariant=Disabled  NCopyVariant=Disabled_SignalSpec  FilterICVariant=Disabled  IntegratorICVariant=InternalICs  ExternalResetVariant=Disabled  TRSumVariant=Passthrough  SumFdbkVariant=Disabled  SumVariant=Sum_PI  TsampFilterVariant=InternalTs  TsampNgainVariant=Passthrough  TsampIntegralVariant=Disabled_SignalSpec
  PLL (3ph) : powerlib_meascontrol/PLL/PLL (3ph)  Fmin=59.5  Par_Init=[0, 60]  ParK=[180, 3200, 1]  TcD=1e-4  MaxRateChangeFreq=12  FilterCutOffFreq=25  Ts=1e-5  AGC=on
  Subsystem1 : Subsystem
  Sum1 : Sum  Inputs=|+-
  Sum2 : Sum  Inputs=|+-
  Terminator{,1..4} (5 alike) : Terminator
  WL : Subsystem
  WL1 : Subsystem
  abc to dq0 : powerlib_meascontrol/Transformations/abc to dq0  Alignment=90 degrees behind phase A axis
  abc to dq1 : powerlib_meascontrol/Transformations/abc to dq0  Alignment=90 degrees behind phase A axis
  abc to dq2 : powerlib_meascontrol/Transformations/abc to dq0  Alignment=90 degrees behind phase A axis
  constant : Constant  Value=0
  dq0 to abc : powerlib_meascontrol/Transformations/dq0 to abc  Alignment=90 degrees behind phase A axis
  Va : Outport  VectorParamsAs1DForOutWhenUnconnected=off
  Vb : Outport  Port=2  VectorParamsAs1DForOutWhenUnconnected=off
  Vc : Outport  Port=3  VectorParamsAs1DForOutWhenUnconnected=off
  wires:
  abc to dq0/1 -> Discrete Transfer Fcn3/1
  PLL (3ph)/2 -> [wt], abc to dq1/2, abc to dq2/2, abc to dq0/2
  Demux1/1 -> Add/1, Subsystem1/3(Ud)
  L1/1 -> WL/3(L), WL1/3(L)
  WL/1(Out1) -> Add/3
  [freq] -> WL1/2(freq), WL/2(freq)
  PLL (3ph)/1 -> [freq]
  Demux2/1 -> Va/1
  Add/1 -> Mux/1
  PID Controller2/1 -> Add1/2
  Demux2/2 -> Vb/1
  WL1/1(Out1) -> Add1/3
  Demux1/2 -> Add1/1
  Add1/1 -> Mux/2
  Mux/1 -> dq0 to abc/1
  Demux2/3 -> Vc/1
  dq0 to abc/1 -> Demux2/1
  Subsystem1/1(Id_ref) -> Sum1/1
  PID Controller1/1 -> Add/2
  [wt] -> dq0 to abc/2
  Subsystem1/2(Iq_ref) -> Sum2/1
  Demux1/3 -> Terminator/1
  Demux/3 -> Terminator1/1
  constant/1 -> Mux/3
  IFabcp/1 -> abc to dq2/1
  abc to dq2/1 -> Discrete Transfer Fcn4/1
  Demux3/3 -> Terminator2/1
  Demux3/2 -> Sum2/2, WL/1(In1)
  Demux3/1 -> Sum1/2, WL1/1(In1)
  Sum1/1 -> PID Controller1/1
  Sum2/1 -> PID Controller2/1
  P_set/1 -> Subsystem1/1(P_ref)
  Q_set/1 -> Subsystem1/2(Q_ref)
  Discrete Transfer Fcn3/1 -> Demux/1
  Discrete Transfer Fcn4/1 -> Demux3/1
  Demux/1 -> Terminator3/1
  Demux/2 -> Terminator4/1
  Discrete Transfer Fcn1/1 -> Demux1/1
  Iabcp/1 -> abc to dq0/1
  Vabcp/1 -> abc to dq1/1, PLL (3ph)/1
  abc to dq1/1 -> Discrete Transfer Fcn1/1

== system IEEE39_IBR_FrequencyControl_Fullversion_2020a/G1_GFL/PV_PQ3/Freq_Droop/Subsystem ==
  Dw : Inport
  w : Inport  Port=2
  Add1 : Sum
  Add2 : Sum  Inputs=+++
  Add3 : Sum  Inputs=-+
  Gain : Gain  Gain=eps_u
  Gain1 : Gain  Gain=eps_ps
  Gain2 : Gain  Gain=c(1)
  Gain3 : Gain  Gain=alpha
  Integrator : Integrator  ExternalReset=rising  ZeroCross=off
  Integrator1 : Integrator  ExternalReset=rising  ZeroCross=off
  Saturation : Saturate  UpperLimit=IBR_data(1,6)-IBR_data(1,10)  LowerLimit=IBR_data(1,6)-IBR_data(1,9)
  Scope : Scope  NumInputPorts=3
  Step : Step  Time=3  SampleTime=0
  Step1 : Step  Time=3  SampleTime=0
  delatPset : Outport
  wires:
  Gain2/1 -> Scope/1, Add2/1
  Integrator1/1 -> delatPset/1, Add3/1, Add1/1, Gain2/1
  Step/1 -> Integrator1/2
  Step1/1 -> Integrator/2
  Integrator/1 -> Gain/1
  Gain/1 -> Scope/3, Add2/2
  Dw/1 -> Integrator/1
  Gain1/1 -> Integrator1/1
  Add2/1 -> Gain3/1
  Gain3/1 -> Add1/2
  Add1/1 -> Saturation/1
  Saturation/1 -> Add3/2
  Add3/1 -> Gain1/1
  w/1 -> Scope/2, Add2/3

== system IEEE39_IBR_FrequencyControl_Fullversion_2020a/G1_GFL/PV_PQ3/Subsystem2/Subsystem1 ==
  P_ref : Inport
  Q_ref : Inport  Port=2
  Ud : Inport  Port=3
  Divide5 : Product  Inputs=*/
  Divide6 : Product  Inputs=*/
  Gain1 : Gain  Gain=-2/3
  Gain2 : Gain  Gain=2/3
  Id_ref : Outport  VectorParamsAs1DForOutWhenUnconnected=off
  Iq_ref : Outport  Port=2  VectorParamsAs1DForOutWhenUnconnected=off
  wires:
  Q_ref/1 -> Divide6/1
  Divide6/1 -> Gain1/1
  P_ref/1 -> Divide5/1
  Gain1/1 -> Iq_ref/1
  Divide5/1 -> Gain2/1
  Gain2/1 -> Id_ref/1
  Ud/1 -> Divide6/2, Divide5/2

== system IEEE39_IBR_FrequencyControl_Fullversion_2020a/G1_GFL/PV_PQ3/Subsystem2/WL ==
  In1 : Inport
  freq : Inport  Port=2
  L : Inport  Port=3
  2pai : Constant  Value=2*pi
  Product : Product  Inputs=**
  Product1 : Product  Inputs=***
  Out1 : Outport  VectorParamsAs1DForOutWhenUnconnected=off
  wires:
  2pai/1 -> Product/2
  L/1 -> Product1/3
  freq/1 -> Product/1
  Product1/1 -> Out1/1
  Product/1 -> Product1/2
  In1/1 -> Product1/1

== system IEEE39_IBR_FrequencyControl_Fullversion_2020a/G1_GFL/PV_PQ3/Subsystem2/WL1 ==
  In1 : Inport
  freq : Inport  Port=2
  L : Inport  Port=3
  2pai : Constant  Value=2*pi
  Product : Product
  Product1 : Product  Inputs=3
  Out1 : Outport  VectorParamsAs1DForOutWhenUnconnected=off
  wires:
  2pai/1 -> Product/2
  L/1 -> Product1/3
  freq/1 -> Product/1
  Product1/1 -> Out1/1
  Product/1 -> Product1/2
  In1/1 -> Product1/1

== system IEEE39_IBR_FrequencyControl_Fullversion_2020a/G2_GFL/PV_PQ3/Freq_Droop/Subsystem ==
  Dw : Inport
  w : Inport  Port=2
  Add1 : Sum
  Add2 : Sum  Inputs=+++
  Add3 : Sum  Inputs=-+
  Gain : Gain  Gain=eps_u
  Gain1 : Gain  Gain=eps_ps
  Gain2 : Gain  Gain=c(2)
  Gain3 : Gain  Gain=alpha
  Integrator : Integrator  ExternalReset=rising  ZeroCross=off
  Integrator1 : Integrator  ExternalReset=rising  ZeroCross=off
  Saturation : Saturate  UpperLimit=IBR_data(2,6)-IBR_data(2,10)  LowerLimit=IBR_data(2,6)-IBR_data(2,9)
  Step : Step  Time=3  SampleTime=0
  Step1 : Step  Time=3  SampleTime=0
  delatPset : Outport
  wires:
  w/1 -> Add2/3
  Gain2/1 -> Add2/1
  Integrator1/1 -> delatPset/1, Add3/1, Add1/1, Gain2/1
  Step/1 -> Integrator1/2
  Step1/1 -> Integrator/2
  Integrator/1 -> Gain/1
  Gain/1 -> Add2/2
  Dw/1 -> Integrator/1
  Gain1/1 -> Integrator1/1
  Add2/1 -> Gain3/1
  Gain3/1 -> Add1/2
  Add1/1 -> Saturation/1
  Saturation/1 -> Add3/2
  Add3/1 -> Gain1/1

== system IEEE39_IBR_FrequencyControl_Fullversion_2020a/G2_GFL/PV_PQ3/Subsystem2/Subsystem1 ==
  P_ref : Inport
  Q_ref : Inport  Port=2
  Ud : Inport  Port=3
  Divide5 : Product  Inputs=*/
  Divide6 : Product  Inputs=*/
  Gain1 : Gain  Gain=-2/3
  Gain2 : Gain  Gain=2/3
  Id_ref : Outport  VectorParamsAs1DForOutWhenUnconnected=off
  Iq_ref : Outport  Port=2  VectorParamsAs1DForOutWhenUnconnected=off
  wires:
  Q_ref/1 -> Divide6/1
  Divide6/1 -> Gain1/1
  P_ref/1 -> Divide5/1
  Gain1/1 -> Iq_ref/1
  Divide5/1 -> Gain2/1
  Gain2/1 -> Id_ref/1
  Ud/1 -> Divide6/2, Divide5/2

== system IEEE39_IBR_FrequencyControl_Fullversion_2020a/G2_GFL/PV_PQ3/Subsystem2/WL ==
  In1 : Inport
  freq : Inport  Port=2
  L : Inport  Port=3
  2pai : Constant  Value=2*pi
  Product : Product  Inputs=**
  Product1 : Product  Inputs=***
  Out1 : Outport  VectorParamsAs1DForOutWhenUnconnected=off
  wires:
  2pai/1 -> Product/2
  L/1 -> Product1/3
  freq/1 -> Product/1
  Product1/1 -> Out1/1
  Product/1 -> Product1/2
  In1/1 -> Product1/1

== system IEEE39_IBR_FrequencyControl_Fullversion_2020a/G2_GFL/PV_PQ3/Subsystem2/WL1 ==
  In1 : Inport
  freq : Inport  Port=2
  L : Inport  Port=3
  2pai : Constant  Value=2*pi
  Product : Product
  Product1 : Product  Inputs=3
  Out1 : Outport  VectorParamsAs1DForOutWhenUnconnected=off
  wires:
  2pai/1 -> Product/2
  L/1 -> Product1/3
  freq/1 -> Product/1
  Product1/1 -> Out1/1
  Product/1 -> Product1/2
  In1/1 -> Product1/1

== system IEEE39_IBR_FrequencyControl_Fullversion_2020a/G3_GFL/PV_PQ3/Freq_Droop/Subsystem ==
  Dw : Inport
  w : Inport  Port=2
  Add1 : Sum
  Add2 : Sum  Inputs=+++
  Add3 : Sum  Inputs=-+
  Gain : Gain  Gain=eps_u
  Gain1 : Gain  Gain=eps_ps
  Gain2 : Gain  Gain=c(3)
  Gain3 : Gain  Gain=alpha
  Integrator : Integrator  ExternalReset=rising  ZeroCross=off
  Integrator1 : Integrator  ExternalReset=rising  ZeroCross=off
  Saturation : Saturate  UpperLimit=IBR_data(3,6)-IBR_data(3,10)  LowerLimit=IBR_data(3,6)-IBR_data(3,9)
  Step : Step  Time=3  SampleTime=0
  Step1 : Step  Time=3  SampleTime=0
  delatPset : Outport
  wires:
  w/1 -> Add2/3
  Gain2/1 -> Add2/1
  Integrator1/1 -> delatPset/1, Add3/1, Add1/1, Gain2/1
  Step/1 -> Integrator1/2
  Step1/1 -> Integrator/2
  Integrator/1 -> Gain/1
  Gain/1 -> Add2/2
  Dw/1 -> Integrator/1
  Gain1/1 -> Integrator1/1
  Add2/1 -> Gain3/1
  Gain3/1 -> Add1/2
  Add1/1 -> Saturation/1
  Saturation/1 -> Add3/2
  Add3/1 -> Gain1/1

== system IEEE39_IBR_FrequencyControl_Fullversion_2020a/G3_GFL/PV_PQ3/Subsystem2/Subsystem1 ==
  P_ref : Inport
  Q_ref : Inport  Port=2
  Ud : Inport  Port=3
  Divide5 : Product  Inputs=*/
  Divide6 : Product  Inputs=*/
  Gain1 : Gain  Gain=-2/3
  Gain2 : Gain  Gain=2/3
  Id_ref : Outport  VectorParamsAs1DForOutWhenUnconnected=off
  Iq_ref : Outport  Port=2  VectorParamsAs1DForOutWhenUnconnected=off
  wires:
  Q_ref/1 -> Divide6/1
  Divide6/1 -> Gain1/1
  P_ref/1 -> Divide5/1
  Gain1/1 -> Iq_ref/1
  Divide5/1 -> Gain2/1
  Gain2/1 -> Id_ref/1
  Ud/1 -> Divide6/2, Divide5/2

== system IEEE39_IBR_FrequencyControl_Fullversion_2020a/G3_GFL/PV_PQ3/Subsystem2/WL ==
  In1 : Inport
  freq : Inport  Port=2
  L : Inport  Port=3
  2pai : Constant  Value=2*pi
  Product : Product  Inputs=**
  Product1 : Product  Inputs=***
  Out1 : Outport  VectorParamsAs1DForOutWhenUnconnected=off
  wires:
  2pai/1 -> Product/2
  L/1 -> Product1/3
  freq/1 -> Product/1
  Product1/1 -> Out1/1
  Product/1 -> Product1/2
  In1/1 -> Product1/1

== system IEEE39_IBR_FrequencyControl_Fullversion_2020a/G3_GFL/PV_PQ3/Subsystem2/WL1 ==
  In1 : Inport
  freq : Inport  Port=2
  L : Inport  Port=3
  2pai : Constant  Value=2*pi
  Product : Product
  Product1 : Product  Inputs=3
  Out1 : Outport  VectorParamsAs1DForOutWhenUnconnected=off
  wires:
  2pai/1 -> Product/2
  L/1 -> Product1/3
  freq/1 -> Product/1
  Product1/1 -> Out1/1
  Product/1 -> Product1/2
  In1/1 -> Product1/1

== system IEEE39_IBR_FrequencyControl_Fullversion_2020a/G4_GFL1/PV_PQ3/Freq_Droop/Subsystem ==
  Dw : Inport
  w : Inport  Port=2
  Add1 : Sum
  Add2 : Sum  Inputs=+++
  Add3 : Sum  Inputs=-+
  Gain : Gain  Gain=eps_u
  Gain1 : Gain  Gain=eps_ps
  Gain2 : Gain  Gain=c(4)
  Gain3 : Gain  Gain=alpha
  Integrator : Integrator  ExternalReset=rising  ZeroCross=off
  Integrator1 : Integrator  ExternalReset=rising  ZeroCross=off
  Saturation : Saturate  UpperLimit=IBR_data(4,6)-IBR_data(4,10)  LowerLimit=IBR_data(4,6)-IBR_data(4,9)
  Step : Step  Time=3  SampleTime=0
  Step1 : Step  Time=3  SampleTime=0
  delatPset : Outport
  wires:
  w/1 -> Add2/3
  Gain2/1 -> Add2/1
  Integrator1/1 -> delatPset/1, Add3/1, Add1/1, Gain2/1
  Step/1 -> Integrator1/2
  Step1/1 -> Integrator/2
  Integrator/1 -> Gain/1
  Gain/1 -> Add2/2
  Dw/1 -> Integrator/1
  Gain1/1 -> Integrator1/1
  Add2/1 -> Gain3/1
  Gain3/1 -> Add1/2
  Add1/1 -> Saturation/1
  Saturation/1 -> Add3/2
  Add3/1 -> Gain1/1

== system IEEE39_IBR_FrequencyControl_Fullversion_2020a/G4_GFL1/PV_PQ3/Subsystem2/Subsystem1 ==
  P_ref : Inport
  Q_ref : Inport  Port=2
  Ud : Inport  Port=3
  Divide5 : Product  Inputs=*/
  Divide6 : Product  Inputs=*/
  Gain1 : Gain  Gain=-2/3
  Gain2 : Gain  Gain=2/3
  Id_ref : Outport  VectorParamsAs1DForOutWhenUnconnected=off
  Iq_ref : Outport  Port=2  VectorParamsAs1DForOutWhenUnconnected=off
  wires:
  Q_ref/1 -> Divide6/1
  Divide6/1 -> Gain1/1
  P_ref/1 -> Divide5/1
  Gain1/1 -> Iq_ref/1
  Divide5/1 -> Gain2/1
  Gain2/1 -> Id_ref/1
  Ud/1 -> Divide6/2, Divide5/2

== system IEEE39_IBR_FrequencyControl_Fullversion_2020a/G4_GFL1/PV_PQ3/Subsystem2/WL ==
  In1 : Inport
  freq : Inport  Port=2
  L : Inport  Port=3
  2pai : Constant  Value=2*pi
  Product : Product  Inputs=**
  Product1 : Product  Inputs=***
  Out1 : Outport  VectorParamsAs1DForOutWhenUnconnected=off
  wires:
  2pai/1 -> Product/2
  L/1 -> Product1/3
  freq/1 -> Product/1
  Product1/1 -> Out1/1
  Product/1 -> Product1/2
  In1/1 -> Product1/1

== system IEEE39_IBR_FrequencyControl_Fullversion_2020a/G4_GFL1/PV_PQ3/Subsystem2/WL1 ==
  In1 : Inport
  freq : Inport  Port=2
  L : Inport  Port=3
  2pai : Constant  Value=2*pi
  Product : Product
  Product1 : Product  Inputs=3
  Out1 : Outport  VectorParamsAs1DForOutWhenUnconnected=off
  wires:
  2pai/1 -> Product/2
  L/1 -> Product1/3
  freq/1 -> Product/1
  Product1/1 -> Out1/1
  Product/1 -> Product1/2
  In1/1 -> Product1/1

== system IEEE39_IBR_FrequencyControl_Fullversion_2020a/G5_GFL/PV_PQ3/Freq_Droop/Subsystem ==
  Dw : Inport
  w : Inport  Port=2
  Add1 : Sum
  Add2 : Sum  Inputs=+++
  Add3 : Sum  Inputs=-+
  Gain : Gain  Gain=eps_u
  Gain1 : Gain  Gain=eps_ps
  Gain2 : Gain  Gain=c(5)
  Gain3 : Gain  Gain=alpha
  Integrator : Integrator  ExternalReset=rising  ZeroCross=off
  Integrator1 : Integrator  ExternalReset=rising  ZeroCross=off
  Saturation : Saturate  UpperLimit=IBR_data(5,6)-IBR_data(5,10)  LowerLimit=IBR_data(5,6)-IBR_data(5,9)
  Step : Step  Time=3  SampleTime=0
  Step1 : Step  Time=3  SampleTime=0
  delatPset : Outport
  wires:
  w/1 -> Add2/3
  Gain2/1 -> Add2/1
  Integrator1/1 -> delatPset/1, Add3/1, Add1/1, Gain2/1
  Step/1 -> Integrator1/2
  Step1/1 -> Integrator/2
  Integrator/1 -> Gain/1
  Gain/1 -> Add2/2
  Dw/1 -> Integrator/1
  Gain1/1 -> Integrator1/1
  Add2/1 -> Gain3/1
  Gain3/1 -> Add1/2
  Add1/1 -> Saturation/1
  Saturation/1 -> Add3/2
  Add3/1 -> Gain1/1

== system IEEE39_IBR_FrequencyControl_Fullversion_2020a/G5_GFL/PV_PQ3/Subsystem2/Subsystem1 ==
  P_ref : Inport
  Q_ref : Inport  Port=2
  Ud : Inport  Port=3
  Divide5 : Product  Inputs=*/
  Divide6 : Product  Inputs=*/
  Gain1 : Gain  Gain=-2/3
  Gain2 : Gain  Gain=2/3
  Id_ref : Outport  VectorParamsAs1DForOutWhenUnconnected=off
  Iq_ref : Outport  Port=2  VectorParamsAs1DForOutWhenUnconnected=off
  wires:
  Q_ref/1 -> Divide6/1
  Divide6/1 -> Gain1/1
  P_ref/1 -> Divide5/1
  Gain1/1 -> Iq_ref/1
  Divide5/1 -> Gain2/1
  Gain2/1 -> Id_ref/1
  Ud/1 -> Divide6/2, Divide5/2

== system IEEE39_IBR_FrequencyControl_Fullversion_2020a/G5_GFL/PV_PQ3/Subsystem2/WL ==
  In1 : Inport
  freq : Inport  Port=2
  L : Inport  Port=3
  2pai : Constant  Value=2*pi
  Product : Product  Inputs=**
  Product1 : Product  Inputs=***
  Out1 : Outport  VectorParamsAs1DForOutWhenUnconnected=off
  wires:
  2pai/1 -> Product/2
  L/1 -> Product1/3
  freq/1 -> Product/1
  Product1/1 -> Out1/1
  Product/1 -> Product1/2
  In1/1 -> Product1/1

== system IEEE39_IBR_FrequencyControl_Fullversion_2020a/G5_GFL/PV_PQ3/Subsystem2/WL1 ==
  In1 : Inport
  freq : Inport  Port=2
  L : Inport  Port=3
  2pai : Constant  Value=2*pi
  Product : Product
  Product1 : Product  Inputs=3
  Out1 : Outport  VectorParamsAs1DForOutWhenUnconnected=off
  wires:
  2pai/1 -> Product/2
  L/1 -> Product1/3
  freq/1 -> Product/1
  Product1/1 -> Out1/1
  Product/1 -> Product1/2
  In1/1 -> Product1/1

== system IEEE39_IBR_FrequencyControl_Fullversion_2020a/G6_GFL/PV_PQ3/Freq_Droop/Subsystem ==
  Dw : Inport
  w : Inport  Port=2
  Add1 : Sum
  Add2 : Sum  Inputs=+++
  Add3 : Sum  Inputs=-+
  Gain : Gain  Gain=eps_u
  Gain1 : Gain  Gain=eps_ps
  Gain2 : Gain  Gain=c(6)
  Gain3 : Gain  Gain=alpha
  Integrator : Integrator  ExternalReset=rising  ZeroCross=off
  Integrator1 : Integrator  ExternalReset=rising  ZeroCross=off
  Saturation : Saturate  UpperLimit=IBR_data(6,6)-IBR_data(6,10)  LowerLimit=IBR_data(6,6)-IBR_data(6,9)
  Step : Step  Time=3  SampleTime=0
  Step1 : Step  Time=3  SampleTime=0
  delatPset : Outport
  wires:
  w/1 -> Add2/3
  Gain2/1 -> Add2/1
  Integrator1/1 -> delatPset/1, Add3/1, Add1/1, Gain2/1
  Step/1 -> Integrator1/2
  Step1/1 -> Integrator/2
  Integrator/1 -> Gain/1
  Gain/1 -> Add2/2
  Dw/1 -> Integrator/1
  Gain1/1 -> Integrator1/1
  Add2/1 -> Gain3/1
  Gain3/1 -> Add1/2
  Add1/1 -> Saturation/1
  Saturation/1 -> Add3/2
  Add3/1 -> Gain1/1

== system IEEE39_IBR_FrequencyControl_Fullversion_2020a/G6_GFL/PV_PQ3/Subsystem2/Subsystem1 ==
  P_ref : Inport
  Q_ref : Inport  Port=2
  Ud : Inport  Port=3
  Divide5 : Product  Inputs=*/
  Divide6 : Product  Inputs=*/
  Gain1 : Gain  Gain=-2/3
  Gain2 : Gain  Gain=2/3
  Id_ref : Outport  VectorParamsAs1DForOutWhenUnconnected=off
  Iq_ref : Outport  Port=2  VectorParamsAs1DForOutWhenUnconnected=off
  wires:
  Q_ref/1 -> Divide6/1
  Divide6/1 -> Gain1/1
  P_ref/1 -> Divide5/1
  Gain1/1 -> Iq_ref/1
  Divide5/1 -> Gain2/1
  Gain2/1 -> Id_ref/1
  Ud/1 -> Divide6/2, Divide5/2
